simulink model "inv_cin2"  (R2020b)
settings: Solver=VariableStepAuto  StartTime=1  StopTime=39  RelTol=1e-3
libraries: simulink x2, roblocks x1
settings Model: PacingRate=3  Creator=beatr  LastModifiedBy=Stefano
settings SolverCC: ZeroCrossAlgorithm=Adaptive
settings DebuggingCC: IgnoredZcDiagnostic=none

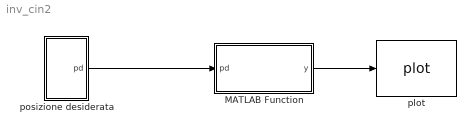
== system inv_cin2 ==
  MATLAB Function : MATLAB Function  TreatAsAtomicUnit=on
  plot : roblocks/Arm/plot  robot=p2  fps=5  holdplot=on
  posizione desiderata : Subsystem
  wires:
  MATLAB Function/1(y) -> plot/1
  posizione desiderata/1(pd) -> MATLAB Function/1(pd)

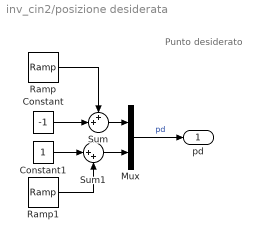
== system inv_cin2/posizione desiderata ==
  note: Punto desiderato
  Constant : Constant  Value=-1
  Constant1 : Constant
  Mux : Mux  Inputs=2
  Ramp : simulink/Sources/Ramp  slope=1/10  start=10  InitialOutput=0
  Ramp1 : simulink/Sources/Ramp  slope=-0.5/10  start=10  InitialOutput=0
  Sum : Sum  Inputs=++|
  Sum1 : Sum  Inputs=|++
  pd : Outport
  wires:
  Constant/1 -> Sum/2
  Mux/1 -> pd/1  "pd"
  Sum/1 -> Mux/1
  Ramp/1 -> Sum/1
  Constant1/1 -> Sum1/1
  Sum1/1 -> Mux/2
  Ramp1/1 -> Sum1/2

== matlab function inv_cin2/MATLAB Function ==
  data: pd input; y output
function y = cinematica_inversa(pd)

a1=1;
a2=1;

y=zeros(2,1);

c2=(pd(1)^2+pd(2)^2-a1^2-a2^2)/(2*a1*a2);

y(2)=acos(c2);


alpha= atan2(pd(2),pd(1));

a=(pd(1)^2+pd(2)^2+a1^2-a2^2)/(2*a1*sqrt(pd(1)^2+pd(2)^2));

beta=acos(a);

y(1)=alpha-beta;
